simulink model "gm_uz_dutycyclemeas"  (R2024a)
settings: Solver=FixedStepDiscrete  StartTime=0.0  StopTime=0.2e-3  RelTol=1e-3
undefined symbols (not defined in the file or in its folder): t_clk, t_clk_sig
libraries: simulink x2, hdlsllib x1
settings Model: Creator=Geiger  LastModifiedBy=Geiger
settings SolverCC: AlgebraicLoopSolver=TrustRegion
settings DataIOCC: LimitDataPoints=on  SaveOutput=off  SaveTime=off
settings OptimizationCC: BlockReduction=off  ConditionallyExecuteInputs=off  DefaultParameterBehavior=Inlined  LifeSpan=inf
settings DebuggingCC: AlgebraicLoopMsg=error  InheritedTsInSrcMsg=none  SingleTaskRateTransMsg=error  UnconnectedInputMsg=warning  UnconnectedOutputMsg=warning  UnconnectedLineMsg=warning  AllowSymbolicDim=off  StrictBusMsg=ErrorOnBusTreatedAsVector  SFUnexpectedBacktrackingDiag=warning  SFNoUnconditionalDefaultTransitionDiag=warning  SFExecutionAtInitializationDiag=none  ArithmeticOperatorsInVariantConditions=warning
settings HardwareCC: ProdBitPerPointer=32  ProdBitPerSizeT=32  ProdBitPerPtrDiffT=32  ProdLargestAtomicFloat=None  ProdIntDivRoundTo=Undefined  ProdEndianess=Unspecified  ProdWordSize=32  ProdHWDeviceType=ASIC/FPGA->ASIC/FPGA  ProdEqTarget=off
settings ModelReferenceCC: EnableRefExpFcnMdlSchedulingChecks=on
settings SFSimCC: SimUseLocalCustomCode=off  CustomCodeUndefinedFunction=UseInterfaceOnly
settings RTWCC: RTWUseLocalCustomCode=off  GPUComputeCapability=3.5
settings CodeAppCC: StateflowObjectComments=on
settings GRTTargetCC: TargetLangStandard=C89/C90 (ANSI)
settings ConfigComp: CovScope=ReferencedModels  CovMetricSettings=dw  CovSaveCumulativeToWorkspaceVar=on  CovSaveSingleToWorkspaceVar=on  CovExternalEMLEnable=off  CovSFcnEnable=off

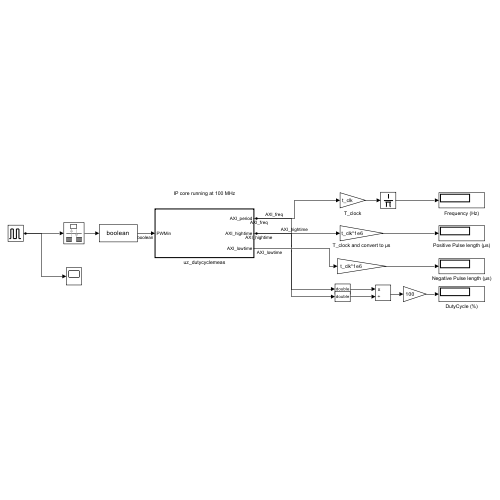
[thumbnail: Simulink's stored preview of the top-level diagram]
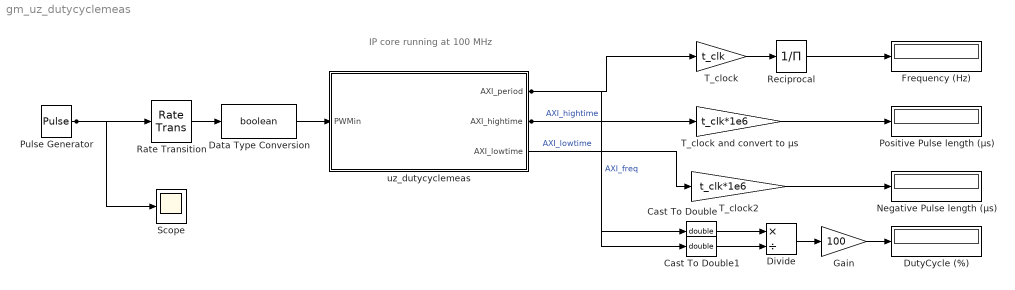
== system gm_uz_dutycyclemeas ==
  note: IP core running at 100 MHz
  Cast To Double : DataTypeConversion  OutDataTypeStr=double  SaturateOnIntegerOverflow=off  RndMeth=Floor
  Cast To Double1 : DataTypeConversion  OutDataTypeStr=double  SaturateOnIntegerOverflow=off  RndMeth=Floor
  Data Type Conversion : DataTypeConversion  OutDataTypeStr=boolean  SaturateOnIntegerOverflow=off  RndMeth=Floor
  Divide : Product  Inputs=*/
  DutyCycle (%) : Display
  Frequency (Hz) : Display
  Gain : Gain  Gain=100
  Negative Pulse length (µs) : Display
  Positive Pulse length (µs) : Display
  Pulse Generator : DiscretePulseGenerator  PulseType=Time based  Period=t_clk_sig  PulseWidth=7.52
  Rate Transition : RateTransition  Deterministic=off  OutPortSampleTime=t_clk
  Reciprocal : Product  Inputs=/
  Scope : Scope
  T_clock : Gain  Gain=t_clk
  T_clock and convert to µs : Gain  Gain=t_clk*1e6
  T_clock2 : Gain  Gain=t_clk*1e6
  uz_dutycyclemeas : Subsystem  TreatAsAtomicUnit=on
  wires:
  Cast To Double1/1 -> Divide/2
  Cast To Double/1 -> Divide/1
  T_clock and convert to µs/1 -> Positive Pulse length (µs)/1
  Divide/1 -> Gain/1
  Rate Transition/1 -> Data Type Conversion/1
  Data Type Conversion/1 -> uz_dutycyclemeas/1(PWMin)
  Pulse Generator/1 -> Rate Transition/1, Scope/1
  uz_dutycyclemeas/1(AXI_period) -> Cast To Double1/1, T_clock/1  "AXI_freq"
  T_clock2/1 -> Negative Pulse length (µs)/1
  T_clock/1 -> Reciprocal/1
  Reciprocal/1 -> Frequency (Hz)/1
  uz_dutycyclemeas/3(AXI_lowtime) -> T_clock2/1  "AXI_lowtime"
  Gain/1 -> DutyCycle (%)/1
  uz_dutycyclemeas/2(AXI_hightime) -> T_clock and convert to µs/1, Cast To Double/1  "AXI_hightime"

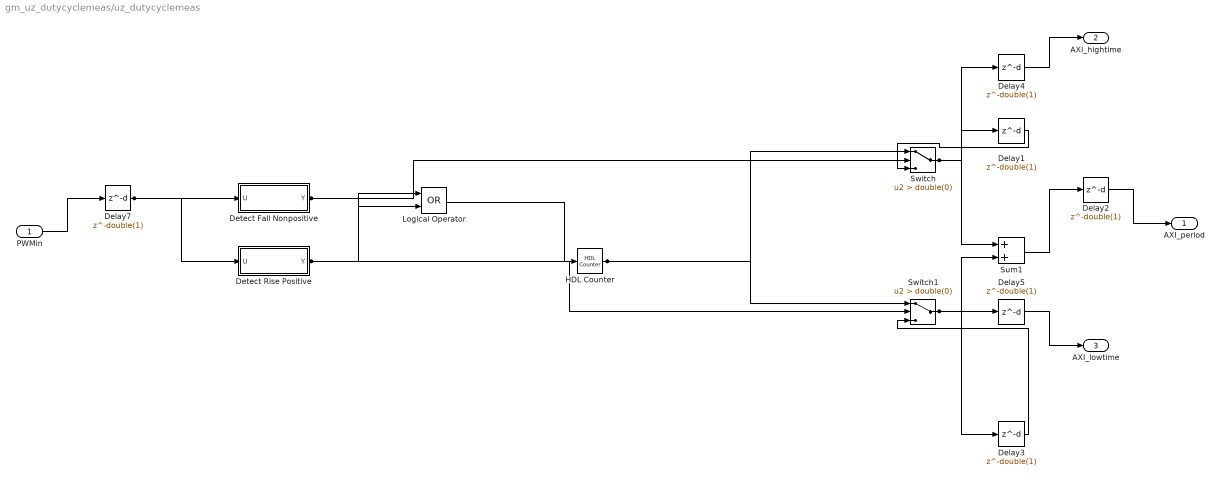
== system gm_uz_dutycyclemeas/uz_dutycyclemeas ==
  PWMin : Inport  OutDataTypeStr=boolean  PortDimensions=1  SampleTime=1e-08
  Delay{1..5,7} (6 alike) : Delay  DelayLength=double(1)  InitialCondition=0  SampleTime=1e-08
  Detect Fall Nonpositive : Subsystem  mask(Detect Fall Nonpositive){vinit=double(0), InputProcessing=Elements as channels (sample based), OutDataTypeStr=boolean}
      mask prompts: vinit "Simulink:masks:InitialCondition_MP"; InputProcessing "Simulink:masks:InputProcessing_MP"; OutDataTypeStr "Simulink:masks:OutputDataType_MP"
      mask help: Simulink:masks:DetectFallNonpositive_MD
      mask init:
      | InputProcessing = 'Elements as channels (sample based)';
      | OutDataTypeStr = 'boolean';
      | vinit = double(0);
      mask TypeOptions InputProcessing: Simulink:masks:ColumnsAsChannelsFrameBased | Simulink:masks:ElementsAsChannelsSampleBased
      mask TypeOptions OutDataTypeStr: Simulink:masks:uint8 | Simulink:masks:boolean
      mask Display: fprintf('U <= 0\n&  NOT\nU/z <= 0')
  Detect Rise Positive : Subsystem  mask(Detect Rise Positive){vinit=double(0), InputProcessing=Elements as channels (sample based), OutDataTypeStr=boolean}
      mask prompts: vinit "Simulink:masks:InitialCondition_MP"; InputProcessing "Simulink:masks:InputProcessing_MP"; OutDataTypeStr "Simulink:masks:OutputDataType_MP"
      mask help: Simulink:masks:DetectRisePositive_MD
      mask init:
      | InputProcessing = 'Elements as channels (sample based)';
      | OutDataTypeStr = 'boolean';
      | vinit = double(0);
      mask TypeOptions InputProcessing: Simulink:masks:ColumnsAsChannelsFrameBased | Simulink:masks:ElementsAsChannelsSampleBased
      mask TypeOptions OutDataTypeStr: Simulink:masks:uint8 | Simulink:masks:boolean
      mask Display: fprintf('U > 0\n&  NOT\nU/z > 0')
  HDL Counter : hdlsllib/Sources/HDL Counter  CountType=Count limited  CountInit=1  CountStep=1  CountMax=2500000  CountFromType=Specify  CountFrom=1  CountResetPort=on  CountLoadPort=off  CountEnbPort=off  CountDirPort=off  CountHitOutputPort=off  CountDataType=Unsigned  CountWordLen=32  CountFracLen=0  CountSampTime=1
  Logical Operator : Logic  Operator=OR  AllPortsSameDT=off  OutDataTypeStr=boolean  SampleTime=1e-08
  Sum1 : Sum  OutDataTypeStr=uint32  AccumDataTypeStr=uint32  SampleTime=1e-08
  Switch : Switch  Criteria=u2 > Threshold  Threshold=double(0)  OutDataTypeStr=uint32  SampleTime=1e-08  SaturateOnIntegerOverflow=off  InputSameDT=off
  Switch1 : Switch  Criteria=u2 > Threshold  Threshold=double(0)  OutDataTypeStr=uint32  SampleTime=1e-08  SaturateOnIntegerOverflow=off  InputSameDT=off
  AXI_period : Outport  SampleTime=1e-08  VectorParamsAs1DForOutWhenUnconnected=off
  AXI_hightime : Outport  Port=2  SampleTime=1e-08  VectorParamsAs1DForOutWhenUnconnected=off
  AXI_lowtime : Outport  Port=3  SampleTime=1e-08  VectorParamsAs1DForOutWhenUnconnected=off
  wires:
  PWMin/1 -> Delay7/1
  Delay1/1 -> Switch/3
  Delay2/1 -> AXI_period/1
  Delay3/1 -> Switch1/3
  Delay4/1 -> AXI_hightime/1
  Delay5/1 -> AXI_lowtime/1
  Delay7/1 -> Detect Fall Nonpositive/1(U), Detect Rise Positive/1(U)
  Detect Fall Nonpositive/1(Y) -> Switch/2, Logical Operator/2
  Detect Rise Positive/1(Y) -> Switch1/2, Logical Operator/1
  HDL Counter/1 -> Switch1/1, Switch/1
  Logical Operator/1 -> HDL Counter/1
  Sum1/1 -> Delay2/1
  Switch/1 -> Sum1/1, Delay4/1, Delay1/1
  Switch1/1 -> Sum1/2, Delay5/1, Delay3/1

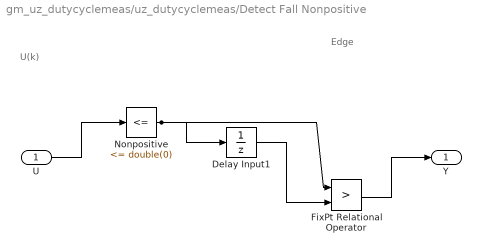
== system gm_uz_dutycyclemeas/uz_dutycyclemeas/Detect Fall Nonpositive ==
  note: U(k)
  note: Edge
  U : Inport  OutDataTypeStr=boolean  SampleTime=1e-08
  Delay Input1 : UnitDelay  SampleTime=1e-08
  FixPt Relational Operator : RelationalOperator  Operator=>  OutDataTypeStr=boolean  SampleTime=1e-08  InputSameDT=off
  Nonpositive : simulink/Logic and Bit Operations/Compare To Constant  relop=<=  const=double(0)  OutDataTypeStr=boolean
  Y : Outport  SampleTime=1e-08
  wires:
  U/1 -> Nonpositive/1
  Delay Input1/1 -> FixPt Relational Operator/2
  FixPt Relational Operator/1 -> Y/1
  Nonpositive/1 -> FixPt Relational Operator/1, Delay Input1/1

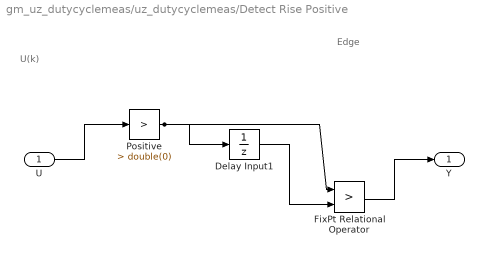
== system gm_uz_dutycyclemeas/uz_dutycyclemeas/Detect Rise Positive ==
  note: U(k)
  note: Edge
  U : Inport  OutDataTypeStr=boolean  SampleTime=1e-08
  Delay Input1 : UnitDelay  SampleTime=1e-08
  FixPt Relational Operator : RelationalOperator  Operator=>  OutDataTypeStr=boolean  SampleTime=1e-08  InputSameDT=off
  Positive : simulink/Logic and Bit Operations/Compare To Constant  relop=>  const=double(0)  OutDataTypeStr=boolean
  Y : Outport  SampleTime=1e-08
  wires:
  U/1 -> Positive/1
  Delay Input1/1 -> FixPt Relational Operator/2
  FixPt Relational Operator/1 -> Y/1
  Positive/1 -> FixPt Relational Operator/1, Delay Input1/1
